simulink model "TSFS06Lab3"  (Simulink 8.2)
settings: Solver=ode23tb  SolverMode=SingleTasking  StartTime=0.0  StopTime=40  RelTol=1e-3  AbsTol=1e-6
values from neighbouring files (symbols this model uses):
  h1Init = Uref(1,1)    [labbskal.m]
  Jnorm = norminv(1-pfa/2,my,std_res)    [labbskal.m]
undefined symbols (not defined in the file or in its folder): d1, d2, d3, d4, watertankparams
undefined symbols (not defined in the file): faults
libraries: simulink x21, simulink_need_slupdate x1
settings Model: Creator=klein  LastModifiedBy=adalu838  ExtModeTrigMode=oneshot  ExtModeArmWhenConnect=off  ExtModeAutoUpdateStatusClock=off
settings DataIOCC: LimitDataPoints=off
settings OptimizationCC: BlockReduction=off  BooleanDataType=off  InitFltsAndDblsToZero=on
settings DebuggingCC: SaveWithParameterizedLinksMsg=none  SignalResolutionControl=TryResolveAllWithWarning  SolverPrmCheckMsg=none  MultiTaskDSMMsg=warning  MultiTaskCondExecSysMsg=none
settings HardwareCC: TargetUnknown=on
settings RTWCC: IncludeERTFirstTime=on

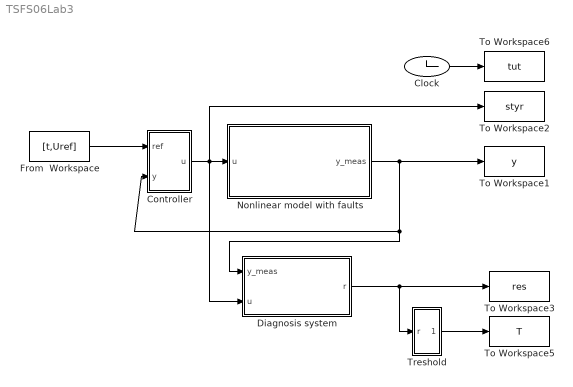
== system TSFS06Lab3 ==
  Clock : Clock
  Controller : Subsystem
  Diagnosis system : Subsystem
  From  Workspace : FromWorkspace  VariableName=[t,Uref]  SampleTime=0.1
  Nonlinear model with faults : Subsystem  mask(Nonlinear WTmodel with faults){fa=faults(1), fs=faults(2:5), fl=faults(6:8), fc=faults(9:10), tstep=15, traise=2, noise=on}
      mask prompts: fa "Actuator faults fa"; fs "SensorFaults fs=[fh1 fh2 ff1 ff2]"; fl "Leaks fl=[fl1 fl2 fl3]"; fc "Clogging fc=[fc1 fc2]"; tstep "Fault initialization time"; traise "Fault ramp duration"; noise "Measurement noise"
  To Workspace1 : ToWorkspace  VariableName=y  SampleTime=0.1
  To Workspace2 : ToWorkspace  VariableName=styr  SampleTime=0.1
  To Workspace3 : ToWorkspace  VariableName=res  SampleTime=0.1
  To Workspace5 : ToWorkspace  VariableName=T  SampleTime=0.1
  To Workspace6 : ToWorkspace  VariableName=tut  SampleTime=0.1
  Treshold : Subsystem
  wires:
  Treshold/1(d) -> To Workspace5/1
  Diagnosis system/1(r) -> Treshold/1(r), To Workspace3/1
  From  Workspace/1 -> Controller/1(ref)
  Controller/1(u) -> Diagnosis system/2(u), To Workspace2/1, Nonlinear model with faults/1(u)
  Clock/1 -> To Workspace6/1
  Nonlinear model with faults/1(y_meas) -> To Workspace1/1, Controller/2(y), Diagnosis system/1(y_meas)

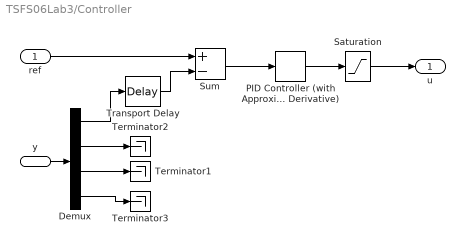
== system TSFS06Lab3/Controller ==
  ref : Inport
  y : Inport  Port=2
  Demux : Demux
  PID Controller (with Approximate Derivative) : simulink_need_slupdate/PID Controller (with Approximate Derivative)  P=10  I=4  D=0  N=100
  Saturation : Saturate  UpperLimit=10  LowerLimit=0  SampleTime=0.1
  Sum : Sum  Inputs=+-  SaturateOnIntegerOverflow=on  InputSameDT=on  OutDataTypeStr=Inherit: Same as first input
  Terminator1 : Terminator
  Terminator2 : Terminator
  Terminator3 : Terminator
  Transport Delay : TransportDelay  DelayTime=0.1  InitialOutput=h1Init
  u : Outport
  wires:
  Demux/3 -> Terminator1/1
  Demux/2 -> Terminator2/1
  y/1 -> Demux/1
  Demux/4 -> Terminator3/1
  ref/1 -> Sum/1
  Sum/1 -> PID Controller (with Approximate Derivative)/1
  PID Controller (with Approximate Derivative)/1 -> Saturation/1
  Saturation/1 -> u/1
  Demux/1 -> Transport Delay/1
  Transport Delay/1 -> Sum/2

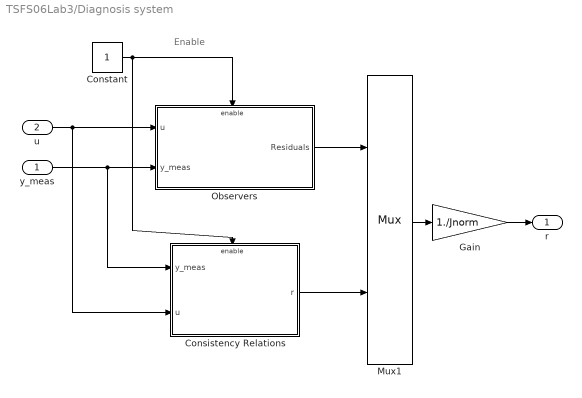
== system TSFS06Lab3/Diagnosis system ==
  note: Enable
  y_meas : Inport
  u : Inport  Port=2
  Consistency Relations : Subsystem
  Constant : Constant
  Gain : Gain  Gain=1./Jnorm  SaturateOnIntegerOverflow=on  OutDataTypeStr=Inherit: Same as input  ParamDataTypeStr=Inherit: Same as input
  Mux1 : Mux  Inputs=2
  Observers : Subsystem
  r : Outport
  wires:
  y_meas/1 -> Observers/2(y_meas), Consistency Relations/1(y_meas)
  u/1 -> Observers/1(u), Consistency Relations/2(u)
  Consistency Relations/1(r) -> Mux1/2
  Observers/1(Residuals) -> Mux1/1
  Mux1/1 -> Gain/1
  Gain/1 -> r/1
  Constant/1 -> Observers/Enable, Consistency Relations/Enable

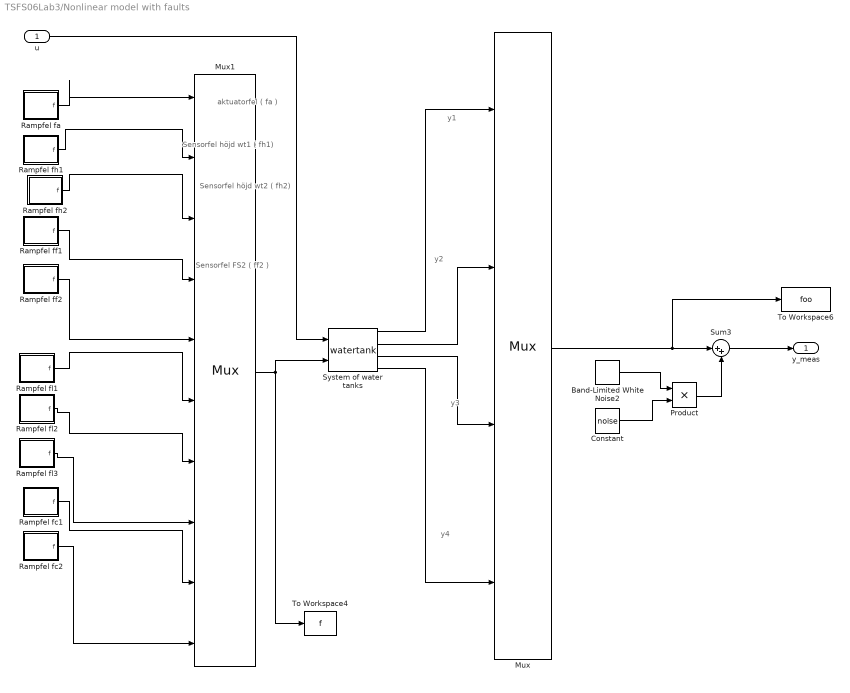
== system TSFS06Lab3/Nonlinear model with faults ==
  note: aktuatorfel ( fa )
  note: Sensorfel höjd wt1 ( fh1)
  note: Sensorfel höjd wt2 ( fh2)
  note: Sensorfel FS2 ( ff2 )
  note: y1
  note: y2
  note: y4
  note: y3
  u : Inport
  Band-Limited White Noise2 : simulink/Sources/Band-Limited White Noise  Cov=NoiseCov  Ts=0.1  seed=NoiseSeed
  Constant : Constant  Value=noise
  Mux : Mux
  Mux1 : Mux  Inputs=10
  Product : Product  RndMeth=Zero
  Rampfel fa : Subsystem  mask(Ramp fault){traise=traise, tstep=tstep, fault=fa}
      mask prompts: traise "Fault ramp duration"; tstep "Fault initiation time"; fault "Fault size"
  Rampfel fc1 : Subsystem  mask(Ramp fault){traise=traise, tstep=tstep, fault=fc(1)}
      mask prompts: traise "Fault ramp duration"; tstep "Fault initiation time"; fault "Fault size"
  Rampfel fc2 : Subsystem  mask(Ramp fault){traise=traise, tstep=tstep, fault=fc(2)}
      mask prompts: traise "Fault ramp duration"; tstep "Fault initiation time"; fault "Fault size"
  Rampfel ff1 : Subsystem  mask(Ramp fault){traise=traise, tstep=tstep, fault=fs(3)}
      mask prompts: traise "Fault ramp duration"; tstep "Fault initiation time"; fault "Fault size"
  Rampfel ff2 : Subsystem  mask(Ramp fault){traise=traise, tstep=tstep, fault=fs(4)}
      mask prompts: traise "Fault ramp duration"; tstep "Fault initiation time"; fault "Fault size"
  Rampfel fh1 : Subsystem  mask(Ramp fault){traise=traise, tstep=tstep, fault=fs(1)}
      mask prompts: traise "Fault ramp duration"; tstep "Fault initiation time"; fault "Fault size"
  Rampfel fh2 : Subsystem  mask(Ramp fault){traise=traise, tstep=tstep, fault=fs(2)}
      mask prompts: traise "Fault ramp duration"; tstep "Fault initiation time"; fault "Fault size"
  Rampfel fl1 : Subsystem  mask(Ramp fault){traise=traise, tstep=tstep, fault=fl(1)}
      mask prompts: traise "Fault ramp duration"; tstep "Fault initiation time"; fault "Fault size"
  Rampfel fl2 : Subsystem  mask(Ramp fault){traise=traise, tstep=tstep, fault=fl(2)}
      mask prompts: traise "Fault ramp duration"; tstep "Fault initiation time"; fault "Fault size"
  Rampfel fl3 : Subsystem  mask(Ramp fault){traise=traise, tstep=tstep, fault=fl(3)}
      mask prompts: traise "Fault ramp duration"; tstep "Fault initiation time"; fault "Fault size"
  Sum3 : Sum  Inputs=|++  SaturateOnIntegerOverflow=on  InputSameDT=on  OutDataTypeStr=Inherit: Same as first input
  System of water tanks : M-S-Function  FunctionName=watertank  Parameters=watertankparams
  To Workspace4 : ToWorkspace  VariableName=f  SampleTime=0.1
  To Workspace6 : ToWorkspace  VariableName=foo  SampleTime=0.1
  y_meas : Outport
  wires:
  Rampfel fc1/1(f) -> Mux1/9
  Rampfel fc2/1(f) -> Mux1/10
  Rampfel fa/1(f) -> Mux1/1
  Rampfel fh1/1(f) -> Mux1/2
  Rampfel fh2/1(f) -> Mux1/3
  Rampfel ff1/1(f) -> Mux1/4
  Rampfel ff2/1(f) -> Mux1/5
  Rampfel fl1/1(f) -> Mux1/6
  Rampfel fl2/1(f) -> Mux1/7
  Rampfel fl3/1(f) -> Mux1/8
  Mux1/1 -> To Workspace4/1, System of water tanks/2
  Mux/1 -> Sum3/1, To Workspace6/1
  Sum3/1 -> y_meas/1
  Constant/1 -> Product/2
  Band-Limited White Noise2/1 -> Product/1
  Product/1 -> Sum3/2
  System of water tanks/1 -> Mux/1
  System of water tanks/2 -> Mux/2
  System of water tanks/3 -> Mux/3
  System of water tanks/4 -> Mux/4
  u/1 -> System of water tanks/1

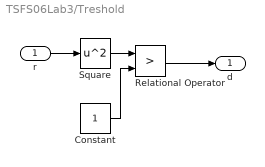
== system TSFS06Lab3/Treshold ==
  r : Inport
  Constant : Constant
  Relational Operator : RelationalOperator  Operator=>  InputSameDT=on
  Square : Math  Operator=square  SaturateOnIntegerOverflow=on
  d : Outport
  wires:
  Relational Operator/1 -> d/1
  Constant/1 -> Relational Operator/2
  Square/1 -> Relational Operator/1
  r/1 -> Square/1

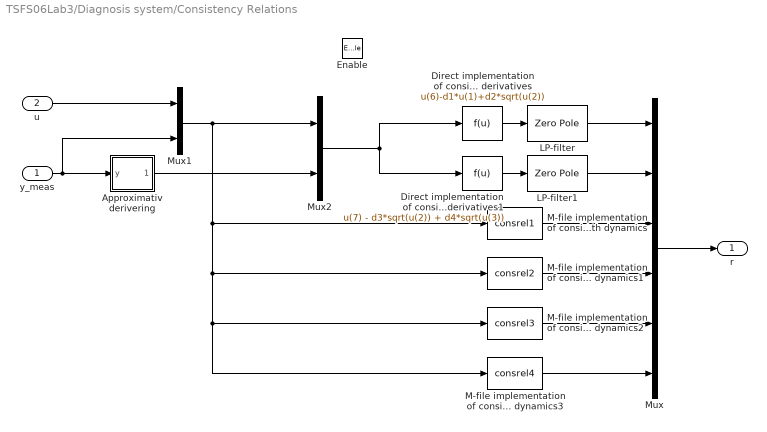
== system TSFS06Lab3/Diagnosis system/Consistency Relations ==
  y_meas : Inport
  u : Inport  Port=2
  Enable : EnablePort
  Approximativ derivering : Subsystem  mask(Approximativ derivering){s=-1}
      mask prompts: s "Pol"
  Direct implementation of consistency relations using approximated derivatives : Fcn  Expr=u(6)-d1*u(1)+d2*sqrt(u(2))
  Direct implementation of consistency relations using approximated derivatives1 : Fcn  Expr=u(7) - d3*sqrt(u(2)) + d4*sqrt(u(3))
  LP-filter : ZeroPole  Zeros=[]  Poles=[-1]
  LP-filter1 : ZeroPole  Zeros=[]  Poles=[-1]
  M-file implementation of consistency relation with dynamics : M-S-Function  FunctionName=consrel1  Parameters=c1params
  M-file implementation of consistency relation with dynamics1 : M-S-Function  FunctionName=consrel2  Parameters=c2params
  M-file implementation of consistency relation with dynamics2 : M-S-Function  FunctionName=consrel3  Parameters=c3params
  M-file implementation of consistency relation with dynamics3 : M-S-Function  FunctionName=consrel4  Parameters=c4params
  Mux : Mux  Inputs=6
  Mux1 : Mux  Inputs=2
  Mux2 : Mux  Inputs=2
  r : Outport
  wires:
  u/1 -> Mux1/1
  y_meas/1 -> Approximativ derivering/1(y), Mux1/2
  Mux/1 -> r/1
  Mux1/1 -> M-file implementation of consistency relation with dynamics3/1, M-file implementation of consistency relation with dynamics2/1, M-file implementation of consistency relation with dynamics1/1, M-file implementation of consistency relation with dynamics/1, Mux2/1
  Approximativ derivering/1(yder) -> Mux2/2
  Direct implementation of consistency relations using approximated derivatives/1 -> LP-filter/1
  Direct implementation of consistency relations using approximated derivatives1/1 -> LP-filter1/1
  LP-filter/1 -> Mux/1
  LP-filter1/1 -> Mux/2
  M-file implementation of consistency relation with dynamics/1 -> Mux/3
  M-file implementation of consistency relation with dynamics1/1 -> Mux/4
  Mux2/1 -> Direct implementation of consistency relations using approximated derivatives/1, Direct implementation of consistency relations using approximated derivatives1/1
  M-file implementation of consistency relation with dynamics2/1 -> Mux/5
  M-file implementation of consistency relation with dynamics3/1 -> Mux/6

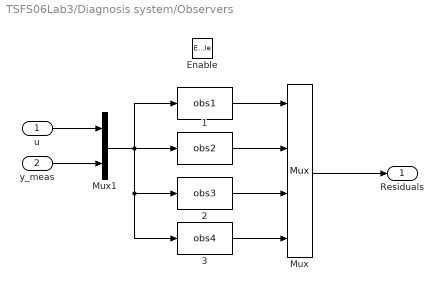
== system TSFS06Lab3/Diagnosis system/Observers ==
  u : Inport
  y_meas : Inport  Port=2
  Enable : EnablePort
  "   " : M-S-Function  FunctionName=obs1  Parameters=obs1params
  "   1" : M-S-Function  FunctionName=obs2  Parameters=obs2params
  "   2" : M-S-Function  FunctionName=obs3  Parameters=obs3params
  "   3" : M-S-Function  FunctionName=obs4  Parameters=obs4params
  Mux : Mux
  Mux1 : Mux  Inputs=2
  Residuals : Outport
  wires:
  Mux/1 -> Residuals/1
  y_meas/1 -> Mux1/2
  Mux1/1 -> "   "/1, "   3"/1, "   2"/1, "   1"/1
  u/1 -> Mux1/1
  "   "/1 -> Mux/1
  "   1"/1 -> Mux/2
  "   2"/1 -> Mux/3
  "   3"/1 -> Mux/4

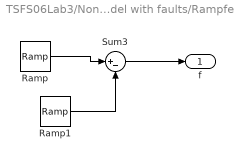
== system TSFS06Lab3/Nonlinear model with faults/Rampfel fa ==
  Ramp : simulink/Sources/Ramp  slope=fault/traise  start=tstep  X0=0
  Ramp1 : simulink/Sources/Ramp  slope=fault/traise  start=tstep+traise  X0=0
  Sum3 : Sum  Inputs=|+-  SaturateOnIntegerOverflow=on  InputSameDT=on  OutDataTypeStr=Inherit: Same as first input
  f : Outport
  wires:
  Ramp/1 -> Sum3/1
  Sum3/1 -> f/1
  Ramp1/1 -> Sum3/2

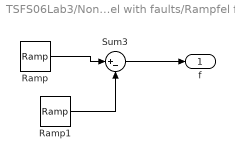
== system TSFS06Lab3/Nonlinear model with faults/Rampfel fc1 ==
  Ramp : simulink/Sources/Ramp  slope=fault/traise  start=tstep  X0=0
  Ramp1 : simulink/Sources/Ramp  slope=fault/traise  start=tstep+traise  X0=0
  Sum3 : Sum  Inputs=|+-  SaturateOnIntegerOverflow=on  InputSameDT=on  OutDataTypeStr=Inherit: Same as first input
  f : Outport
  wires:
  Ramp/1 -> Sum3/1
  Sum3/1 -> f/1
  Ramp1/1 -> Sum3/2

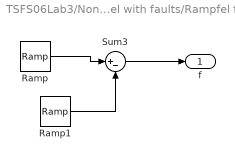
== system TSFS06Lab3/Nonlinear model with faults/Rampfel fc2 ==
  Ramp : simulink/Sources/Ramp  slope=fault/traise  start=tstep  X0=0
  Ramp1 : simulink/Sources/Ramp  slope=fault/traise  start=tstep+traise  X0=0
  Sum3 : Sum  Inputs=|+-  SaturateOnIntegerOverflow=on  InputSameDT=on  OutDataTypeStr=Inherit: Same as first input
  f : Outport
  wires:
  Ramp1/1 -> Sum3/2
  Sum3/1 -> f/1
  Ramp/1 -> Sum3/1

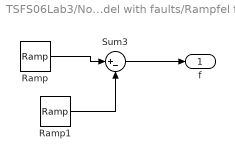
== system TSFS06Lab3/Nonlinear model with faults/Rampfel ff1 ==
  Ramp : simulink/Sources/Ramp  slope=fault/traise  start=tstep  X0=0
  Ramp1 : simulink/Sources/Ramp  slope=fault/traise  start=tstep+traise  X0=0
  Sum3 : Sum  Inputs=|+-  SaturateOnIntegerOverflow=on  InputSameDT=on  OutDataTypeStr=Inherit: Same as first input
  f : Outport
  wires:
  Ramp1/1 -> Sum3/2
  Sum3/1 -> f/1
  Ramp/1 -> Sum3/1

== system TSFS06Lab3/Nonlinear model with faults/Rampfel ff2 ==
  Ramp : simulink/Sources/Ramp  slope=fault/traise  start=tstep  X0=0
  Ramp1 : simulink/Sources/Ramp  slope=fault/traise  start=tstep+traise  X0=0
  Sum3 : Sum  Inputs=|+-  SaturateOnIntegerOverflow=on  InputSameDT=on  OutDataTypeStr=Inherit: Same as first input
  f : Outport
  wires:
  Ramp/1 -> Sum3/1
  Sum3/1 -> f/1
  Ramp1/1 -> Sum3/2

== system TSFS06Lab3/Nonlinear model with faults/Rampfel fh1 ==
  Ramp : simulink/Sources/Ramp  slope=fault/traise  start=tstep  X0=0
  Ramp1 : simulink/Sources/Ramp  slope=fault/traise  start=tstep+traise  X0=0
  Sum3 : Sum  Inputs=|+-  SaturateOnIntegerOverflow=on  InputSameDT=on  OutDataTypeStr=Inherit: Same as first input
  f : Outport
  wires:
  Ramp1/1 -> Sum3/2
  Sum3/1 -> f/1
  Ramp/1 -> Sum3/1

== system TSFS06Lab3/Nonlinear model with faults/Rampfel fh2 ==
  Ramp : simulink/Sources/Ramp  slope=fault/traise  start=tstep  X0=0
  Ramp1 : simulink/Sources/Ramp  slope=fault/traise  start=tstep+traise  X0=0
  Sum3 : Sum  Inputs=|+-  SaturateOnIntegerOverflow=on  InputSameDT=on  OutDataTypeStr=Inherit: Same as first input
  f : Outport
  wires:
  Ramp/1 -> Sum3/1
  Sum3/1 -> f/1
  Ramp1/1 -> Sum3/2

== system TSFS06Lab3/Nonlinear model with faults/Rampfel fl1 ==
  Ramp : simulink/Sources/Ramp  slope=fault/traise  start=tstep  X0=0
  Ramp1 : simulink/Sources/Ramp  slope=fault/traise  start=tstep+traise  X0=0
  Sum3 : Sum  Inputs=|+-  SaturateOnIntegerOverflow=on  InputSameDT=on  OutDataTypeStr=Inherit: Same as first input
  f : Outport
  wires:
  Ramp1/1 -> Sum3/2
  Sum3/1 -> f/1
  Ramp/1 -> Sum3/1

== system TSFS06Lab3/Nonlinear model with faults/Rampfel fl2 ==
  Ramp : simulink/Sources/Ramp  slope=fault/traise  start=tstep  X0=0
  Ramp1 : simulink/Sources/Ramp  slope=fault/traise  start=tstep+traise  X0=0
  Sum3 : Sum  Inputs=|+-  SaturateOnIntegerOverflow=on  InputSameDT=on  OutDataTypeStr=Inherit: Same as first input
  f : Outport
  wires:
  Ramp/1 -> Sum3/1
  Sum3/1 -> f/1
  Ramp1/1 -> Sum3/2

== system TSFS06Lab3/Nonlinear model with faults/Rampfel fl3 ==
  Ramp : simulink/Sources/Ramp  slope=fault/traise  start=tstep  X0=0
  Ramp1 : simulink/Sources/Ramp  slope=fault/traise  start=tstep+traise  X0=0
  Sum3 : Sum  Inputs=|+-  SaturateOnIntegerOverflow=on  InputSameDT=on  OutDataTypeStr=Inherit: Same as first input
  f : Outport
  wires:
  Ramp1/1 -> Sum3/2
  Sum3/1 -> f/1
  Ramp/1 -> Sum3/1

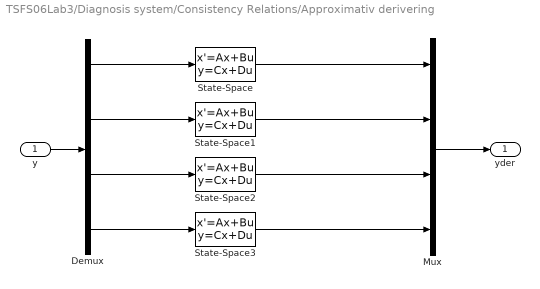
== system TSFS06Lab3/Diagnosis system/Consistency Relations/Approximativ derivering ==
  y : Inport
  Demux : Demux
  Mux : Mux
  State-Space : StateSpace  A=s  B=-s^2  D=-s  X0=s*watertankparams.x0(1)
  State-Space1 : StateSpace  A=s  B=-s^2  D=-s  X0=s*watertankparams.x0(2)
  State-Space2 : StateSpace  A=s  B=-s^2  D=-s  X0=s*watertankparams.d(5)*sqrt(watertankparams.x0(1))
  State-Space3 : StateSpace  A=s  B=-s^2  D=-s  X0=s*watertankparams.d(6)*sqrt(watertankparams.x0(2))
  yder : Outport
  wires:
  y/1 -> Demux/1
  Demux/4 -> State-Space3/1
  Demux/3 -> State-Space2/1
  Demux/2 -> State-Space1/1
  Demux/1 -> State-Space/1
  State-Space/1 -> Mux/1
  State-Space1/1 -> Mux/2
  State-Space2/1 -> Mux/3
  State-Space3/1 -> Mux/4
  Mux/1 -> yder/1
